simulink library "INT_GbxNPos_DD"  (R2016b)
settings: Solver=VariableStepAuto  StartTime=0.0  StopTime=10.0  RelTol=1e-3
settings Model: Creator=bianxuyin  LastModifiedBy=bianxuyin

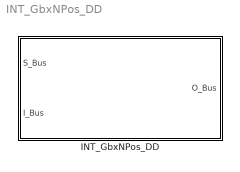
== system INT_GbxNPos_DD ==
  INT_GbxNPos_DD : Subsystem

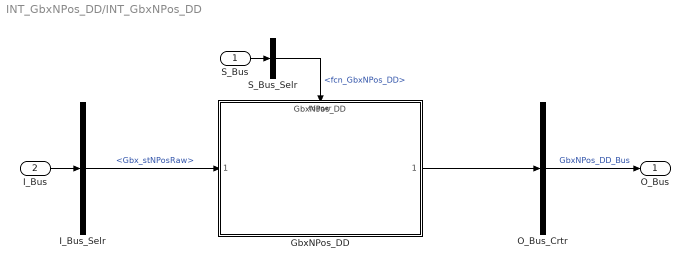
== system INT_GbxNPos_DD/INT_GbxNPos_DD ==
  S_Bus : Inport
  I_Bus : Inport  Port=2
  GbxNPos_DD : ModelReference  ModelNameDialog=GbxNPos_DD  SimulationMode=Normal  ModelReferenceVersion=1.10  TriggerPortName=function  TriggerPortTriggerType=function-call  TriggerPortStatesWhenEnabling=held
  I_Bus_Selr : BusSelector  OutputSignals=Gbx_stNPosRaw
  O_Bus_Crtr : BusCreator  Inputs=1
  S_Bus_Selr : BusSelector  OutputSignals=fcn_GbxNPos_DD
  O_Bus : Outport
  wires:
  S_Bus_Selr/1 -> GbxNPos_DD/Trigger  "<fcn_GbxNPos_DD>"
  S_Bus/1 -> S_Bus_Selr/1
  I_Bus/1 -> I_Bus_Selr/1
  I_Bus_Selr/1 -> GbxNPos_DD/1  "<Gbx_stNPosRaw>"
  O_Bus_Crtr/1 -> O_Bus/1  "GbxNPos_DD_Bus"
  GbxNPos_DD/1 -> O_Bus_Crtr/1
